simulink model "Test3S150Board_QuadDisplay"  (Simulink 6.4)
settings: Solver=ode45  SolverMode=SingleTasking  StartTime=0.0  StopTime=100.0  FixedStep=1  RelTol=1e-3
InitFcn:
  | %% DSPBuilder Start
  | alt_dspbuilder_update_model(bdroot)
  | %% DSPBuilder End
undefined symbols (not defined in the file): Pin_A19, Pin_A20, Pin_AC12, Pin_AE10, Pin_AE12, Pin_AF11, Pin_AH11, Pin_AH8, Pin_AK6, Pin_AL4, Pin_AL5, Pin_AM4, Pin_AM5, Pin_AM6, Pin_AP3, Pin_B19, Pin_C18, Pin_J19, Pin_K19, Pin_L19, Pin_L20
libraries: allblocks_alteradspbuilder2 x17, Stratix_III_EP3SL150_alteradspbuilder2 x5
settings Model: Creator=lkong  LastModifiedBy=lkong
settings DataIOCC: SignalLoggingName=sigsOut
settings OptimizationCC: InlineInvariantSignals=on
settings DebuggingCC: SolverPrmCheckMsg=none  StrictBusMsg=None
settings HardwareCC: TargetUnknown=on
settings GRTTargetCC: ModelReferenceCompliant=off  MatFileLogging=off

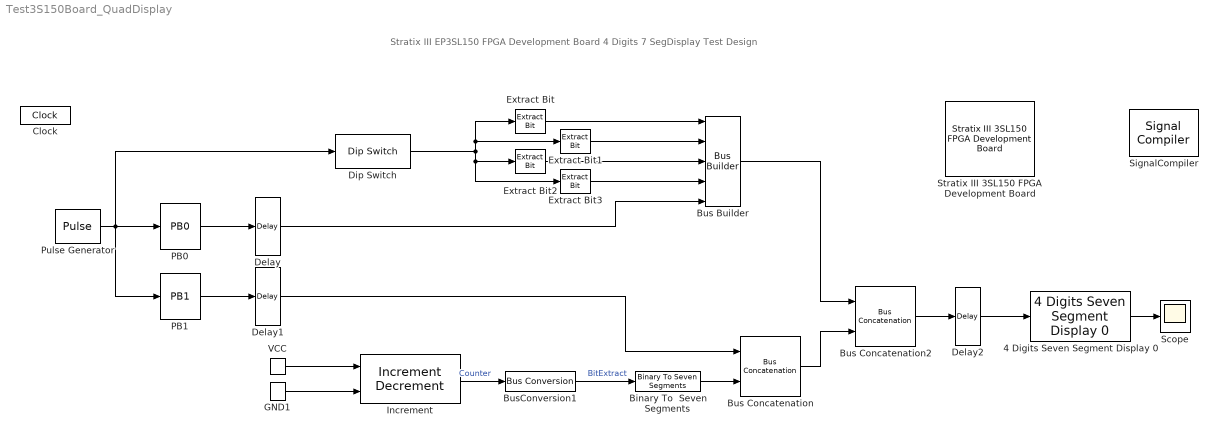
== system Test3S150Board_QuadDisplay ==
  note: Stratix III EP3SL150 FPGA Development Board 4 Digits 7 SegDisplay Test Design
  4 Digits Seven Segment Display 0 : Stratix_III_EP3SL150_alteradspbuilder2/4 Digits Seven Segment Display 0  iofile=d:\ws80\workspace\documentation\designExamples\demos\board\stratixIII_DSPBoard_3S150\tb_Test3S150Board_QuadDisplay\Test3S150Board%5FQuadDisplay_4+Digits+Seven+Segment+Display+0.capture  externalType=Inferred  location=Pin_AE10,Pin_AL5,Pin_AC12,Pin_AM5,Pin_AF11,Pin_AM6,Pin_AP3,Pin_AK6,Pin_AM4,Pin_AE12,Pin_AL4,Pin_AH8,Pin_AH11
  Binary To  Seven Segments : allblocks_alteradspbuilder2/Binary To Seven Segments  pipeline_display=0
  Bus Builder : allblocks_alteradspbuilder2/Bus Builder  BusType=Unsigned Integer  bwl=5  bwr=1  pipeline_display=0
  Bus Concatenation : allblocks_alteradspbuilder2/Bus Concatenation  isSigned=off  awidth=1  bwidth=7  pipeline_display=0
  Bus Concatenation2 : allblocks_alteradspbuilder2/Bus Concatenation  isSigned=off  awidth=5  bwidth=8  pipeline_display=0
  BusConversion1 : allblocks_alteradspbuilder2/Bus Conversion  BusType=Unsigned Integer  ibwl=29  ibwr=0  bwl=4  bwr=0  bitToConnectToOutputLSB=25  round=off  saturate=off  pipeline_display=0
  Clock : allblocks_alteradspbuilder2/Clock  ClockPeriod=10  ClockPeriodUnit=ns  SampleTime=1  SimulationStartCycle=5  PhaseOffset=0  Reset=aclr  ResetType=Active Low  Export=off
  Delay : allblocks_alteradspbuilder2/Delay  pipeline=1  pipeline_display=1  ClockPhase=1  use_ena=off  use_sclr=off  allowFloatingPointOverride=on  logOutputs=off  logFile=d:\ws80\workspace\documentation\designExamples\demos\board\stratixIII_DSPBoard_3S150\tb_Test3S150Board_QuadDisplay\Test3S150Board%5FQuadDisplay_Delay.fixedpointlog  use_init=off  reset_value=1
  Delay1 : allblocks_alteradspbuilder2/Delay  pipeline=1  pipeline_display=1  ClockPhase=1  use_ena=off  use_sclr=off  allowFloatingPointOverride=on  logOutputs=off  logFile=d:\ws80\workspace\documentation\designExamples\demos\board\stratixIII_DSPBoard_3S150\tb_Test3S150Board_QuadDisplay\Test3S150Board%5FQuadDisplay_Delay1.fixedpointlog  use_init=off  reset_value=1
  Delay2 : allblocks_alteradspbuilder2/Delay  pipeline=1  pipeline_display=1  ClockPhase=1  use_ena=off  use_sclr=off  allowFloatingPointOverride=on  logOutputs=off  logFile=d:\ws80\workspace\documentation\designExamples\demos\board\stratixIII_DSPBoard_3S150\tb_Test3S150Board_QuadDisplay\Test3S150Board%5FQuadDisplay_Delay2.fixedpointlog  use_init=off  reset_value=1
  Dip Switch : Stratix_III_EP3SL150_alteradspbuilder2/Dip Switch  iofile=d:\ws80\workspace\documentation\designExamples\demos\board\stratixIII_DSPBoard_3S150\tb_Test3S150Board_QuadDisplay\Test3S150Board%5FQuadDisplay_Dip+Switch.salt  externalType=Inferred  SpecifyClock=off  location=Pin_B19,Pin_A19,Pin_C18,Pin_A20,Pin_K19,Pin_J19,Pin_L19,Pin_L20
  Extract Bit : allblocks_alteradspbuilder2/Extract Bit  BusType=Unsigned Integer  bwl=7  bwr=0  bitToSelect=0  pipeline_display=0
  Extract Bit1 : allblocks_alteradspbuilder2/Extract Bit  BusType=Unsigned Integer  bwl=7  bwr=0  bitToSelect=1  pipeline_display=0
  Extract Bit2 : allblocks_alteradspbuilder2/Extract Bit  BusType=Unsigned Integer  bwl=7  bwr=0  bitToSelect=2  pipeline_display=0
  Extract Bit3 : allblocks_alteradspbuilder2/Extract Bit  BusType=Unsigned Integer  bwl=7  bwr=0  bitToSelect=3  pipeline_display=0
  GND1 : allblocks_alteradspbuilder2/GND  SpecifyClock=off
  Increment : allblocks_alteradspbuilder2/Increment Decrement  BusType=Unsigned Integer  bwl=29  bwr=0  SpecifyClock=off  clr_value=0  direction=Increment  phase_selection=1  use_ena=on  use_sclr=on  pipeline_display=1
  PB0 : Stratix_III_EP3SL150_alteradspbuilder2/PB0  iofile=d:\ws80\workspace\documentation\designExamples\demos\board\stratixIII_DSPBoard_3S150\tb_Test3S150Board_QuadDisplay\Test3S150Board%5FQuadDisplay_PB0.salt  externalType=Inferred  SpecifyClock=off  location=Pin_B17
  PB1 : Stratix_III_EP3SL150_alteradspbuilder2/PB1  iofile=d:\ws80\workspace\documentation\designExamples\demos\board\stratixIII_DSPBoard_3S150\tb_Test3S150Board_QuadDisplay\Test3S150Board%5FQuadDisplay_PB1.salt  externalType=Inferred  SpecifyClock=off  location=Pin_A17
  Pulse Generator : DiscretePulseGenerator  Period=20000  PulseWidth=2
  Scope : Scope
  SignalCompiler : allblocks_alteradspbuilder2/Signal Compiler  DeviceFamily=Stratix III  DeviceName=EP3SL150F1152C4ES  EnableSignalTap=on  SignalTapDepth=512  UseBoardBlock=on  StpUseDefaultClock=on  StpClock=Clock  ExportDir=D:\MATLAB\R2006a\work
  "Stratix III 3SL150 FPGA Development Board " : Stratix_III_EP3SL150_alteradspbuilder2/Stratix III 3SL150 FPGA Development Board   ClockPinIn=Pin_T33  GlobalResetPin=PIN_AP5  device=EP3SL150F1152C4ES
  VCC : allblocks_alteradspbuilder2/VCC  SpecifyClock=off
  wires:
  Pulse Generator/1 -> Dip Switch/1, PB0/1, PB1/1
  GND1/1 -> Increment/2
  VCC/1 -> Increment/1
  Increment/1 -> BusConversion1/1  "Counter"
  BusConversion1/1 -> Binary To  Seven Segments/1  "BitExtract"
  PB0/1 -> Delay/1
  PB1/1 -> Delay1/1
  Bus Concatenation2/1 -> Delay2/1
  Binary To  Seven Segments/1 -> Bus Concatenation/2
  Bus Builder/1 -> Bus Concatenation2/1
  Bus Concatenation/1 -> Bus Concatenation2/2
  Delay/1 -> Bus Builder/5
  Delay1/1 -> Bus Concatenation/1
  Extract Bit/1 -> Bus Builder/1
  Dip Switch/1 -> Extract Bit/1, Extract Bit1/1, Extract Bit2/1, Extract Bit3/1
  Extract Bit1/1 -> Bus Builder/2
  Extract Bit2/1 -> Bus Builder/3
  Extract Bit3/1 -> Bus Builder/4
  Delay2/1 -> 4 Digits Seven Segment Display 0/1
  4 Digits Seven Segment Display 0/1 -> Scope/1
